simulink model "ReactionPendulum_Simulation_Model"  (R2024b)
settings: Solver=ode23  StartTime=0.0  StopTime=T_final  MaxStep=1e-2  RelTol=1e-3
values from neighbouring files (symbols this model uses):
  Control_Gain = 1.3    [PendulumControl_Mamdani_ver2.m]
  fi_pend0 = deg2rad(30)    [PendulumControl_Mamdani_ver2.m]
undefined symbols (not defined in the file or in its folder): fi_dc0, g, J_dc, J_pend, K, kr, kt, omega_dc0, omega_pend0, R_dc, U, uc_dc, uc_pend, uv_dc, uv_pend
libraries: fuzblock x1
settings Model: Creator=Student  LastModifiedBy=Paweł Wiktor
settings SolverCC: ZeroCrossAlgorithm=Adaptive  AlgebraicLoopSolver=TrustRegion
settings DataIOCC: ReturnWorkspaceOutputs=off
settings DebuggingCC: IgnoredZcDiagnostic=none  UnconnectedInputMsg=warning  UnconnectedOutputMsg=warning  UnconnectedLineMsg=warning  ArithmeticOperatorsInVariantConditions=warning
settings ModelReferenceCC: EnableRefExpFcnMdlSchedulingChecks=on
settings SFSimCC: CustomCodeUndefinedFunction=UseInterfaceOnly
settings RTWCC: GPUComputeCapability=3.5

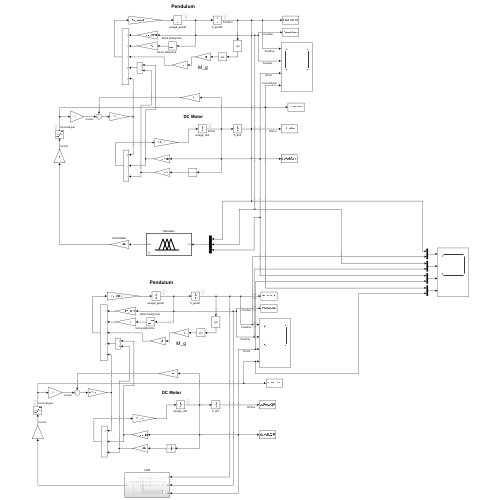
[thumbnail: Simulink's stored preview of the top-level diagram]
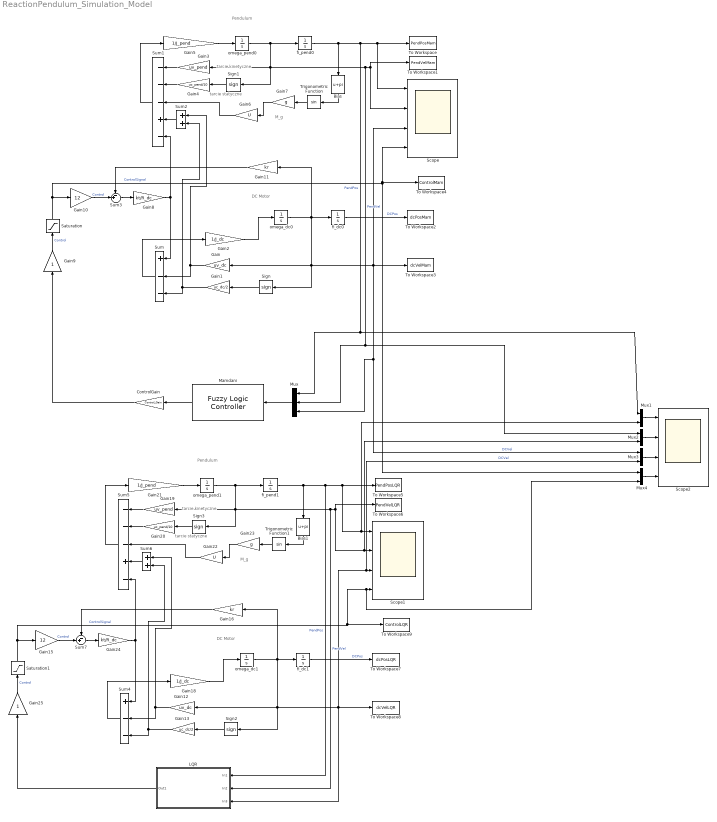
== system ReactionPendulum_Simulation_Model ==
  note: DC Motor
  note: M_g
  note: tarcie kinetyczne
  note: tarcie statyczne
  note: Pendulum
  note: DC Motor
  note: tarcie kinetyczne
  note: Pendulum
  note: tarcie statyczne
  note: M_g
  Bias : Bias  Bias=pi  SaturateOnIntegerOverflow=off
  Bias1 : Bias  Bias=pi  SaturateOnIntegerOverflow=off
  ControlGain : Gain  Gain=Control_Gain
  Gain : Gain  Gain=uv_dc
  Gain1 : Gain  Gain=uc_dc/2
  Gain10 : Gain  Gain=12
  Gain11 : Gain  Gain=kr
  Gain12 : Gain  Gain=uv_dc
  Gain13 : Gain  Gain=uc_dc/2
  Gain15 : Gain  Gain=12
  Gain16 : Gain  Gain=kr
  Gain18 : Gain  Gain=1/J_dc
  Gain19 : Gain  Gain=uv_pend
  Gain2 : Gain  Gain=1/J_dc
  Gain20 : Gain  Gain=uc_pend/10
  Gain21 : Gain  Gain=1/J_pend
  Gain22 : Gain  Gain=U
  Gain23 : Gain  Gain=g
  Gain24 : Gain  Gain=kt/R_dc
  Gain25 : Gain
  Gain3 : Gain  Gain=uv_pend
  Gain4 : Gain  Gain=uc_pend/10
  Gain5 : Gain  Gain=1/J_pend
  Gain6 : Gain  Gain=U
  Gain7 : Gain  Gain=g
  Gain8 : Gain  Gain=kt/R_dc
  Gain9 : Gain
  LQR : Subsystem
  Mamdani : fuzblock/Fuzzy Logic  Controller  FIS=fisMam_ver3  OutputSampleNumber=101  DataType=double  FuzzifiedInputs=off  RuleFiringStrengths=off  RuleOutputs=off  AggregatedOutputs=off  SimulateUsing=Interpreted execution  OutOfRangeInputValueMessage=warning  NoRuleFiredMessage=warning  EmptyOutputFuzzySetMessage=warning
  Mux : Mux  Inputs=3
  Mux{1..4} (4 alike) : Mux  Inputs=2
  Saturation : Saturate  UpperLimit=1  LowerLimit=-1
  Saturation1 : Saturate  UpperLimit=1  LowerLimit=-1
  Scope : Scope  NumInputPorts=4
  Scope1 : Scope  NumInputPorts=4
  Scope2 : Scope  NumInputPorts=4
  Sign{,1..3} (4 alike) : Signum  ZeroCross=off
  Sum : Sum  Inputs=+--
  Sum1 : Sum  Inputs=---+-
  Sum2 : Sum
  Sum3 : Sum  Inputs=-+|
  Sum4 : Sum  Inputs=+--
  Sum5 : Sum  Inputs=---+-
  Sum6 : Sum
  Sum7 : Sum  Inputs=-+|
  To Workspace : ToWorkspace  VariableName=PendPosMam  SaveFormat=Structure With Time  SampleTime=-1
  To Workspace1 : ToWorkspace  VariableName=PendVelMam  SaveFormat=Structure With Time  SampleTime=-1
  To Workspace2 : ToWorkspace  VariableName=dcPosMam  SaveFormat=Structure With Time  SampleTime=-1
  To Workspace3 : ToWorkspace  VariableName=dcVelMam  SaveFormat=Structure With Time  SampleTime=-1
  To Workspace4 : ToWorkspace  VariableName=ControlMam  SaveFormat=Structure With Time  SampleTime=-1
  To Workspace5 : ToWorkspace  VariableName=PendPosLQR  SaveFormat=Structure With Time  SampleTime=-1
  To Workspace6 : ToWorkspace  VariableName=PendVelLQR  SaveFormat=Structure With Time  SampleTime=-1
  To Workspace7 : ToWorkspace  VariableName=dcPosLQR  SaveFormat=Structure With Time  SampleTime=-1
  To Workspace8 : ToWorkspace  VariableName=dcVelLQR  SaveFormat=Structure With Time  SampleTime=-1
  To Workspace9 : ToWorkspace  VariableName=ControlLQR  SaveFormat=Structure With Time  SampleTime=-1
  Trigonometric Function : Trigonometry
  Trigonometric Function1 : Trigonometry
  fi_dc0 : Integrator  InitialCondition=fi_dc0
  fi_dc1 : Integrator  InitialCondition=fi_dc0
  fi_pend0 : Integrator  InitialCondition=fi_pend0
  fi_pend1 : Integrator  InitialCondition=fi_pend0
  omega_dc0 : Integrator  InitialCondition=omega_dc0
  omega_dc1 : Integrator  InitialCondition=omega_dc0
  omega_pend0 : Integrator  InitialCondition=omega_pend0
  omega_pend1 : Integrator  InitialCondition=omega_pend0
  wires:
  Bias/1 -> Trigonometric Function/1
  omega_pend0/1 -> Sign1/1, Mux2/1, Mux/2, To Workspace1/1, Scope/2, Gain3/1, fi_pend0/1  "PendVel"
  Gain4/1 -> Sum1/2
  Sum2/1 -> Sum1/4
  Gain11/1 -> Sum3/1
  Sum/1 -> Gain2/1
  Gain8/1 -> Sum1/5, Sum/1
  Gain3/1 -> Sum1/1
  Trigonometric Function/1 -> Gain7/1
  Sign1/1 -> Gain4/1
  Saturation/1 -> Scope/4, To Workspace4/1, Mux4/1, Gain10/1  "ControlSignal"
  Sign/1 -> Gain1/1
  Gain/1 -> Sum/2, Sum2/1
  Sum1/1 -> Gain5/1
  Gain5/1 -> omega_pend0/1
  Gain1/1 -> Sum/3, Sum2/2
  Gain10/1 -> Sum3/2  "Control"
  Gain6/1 -> Sum1/3
  Sum3/1 -> Gain8/1
  Gain2/1 -> omega_dc0/1
  Gain9/1 -> Saturation/1  "Control"
  fi_dc0/1 -> To Workspace2/1  "DCPos"
  Gain7/1 -> Gain6/1
  Mux/1 -> Mamdani/1
  ControlGain/1 -> Gain9/1
  Mamdani/1 -> ControlGain/1
  fi_pend1/1 -> LQR/1(In1), Mux1/2, Scope1/1, To Workspace5/1, Bias1/1  "PendPos"
  Sum4/1 -> Gain18/1
  Bias1/1 -> Trigonometric Function1/1
  Gain20/1 -> Sum5/2
  Gain25/1 -> Saturation1/1  "Control"
  Trigonometric Function1/1 -> Gain23/1
  Gain18/1 -> omega_dc1/1
  Gain15/1 -> Sum7/2  "Control"
  omega_pend1/1 -> Sign3/1, LQR/2(In2), To Workspace6/1, Mux2/2, Scope1/2, Gain19/1, fi_pend1/1  "PendVel"
  Sum7/1 -> Gain24/1
  Gain21/1 -> omega_pend1/1
  LQR/1(Out1) -> Gain25/1
  Saturation1/1 -> Mux4/2, Scope1/4, To Workspace9/1, Gain15/1  "ControlSignal"
  Gain16/1 -> Sum7/1
  Sum6/1 -> Sum5/4
  Gain12/1 -> Sum4/2, Sum6/1
  Sign2/1 -> Gain13/1
  Gain23/1 -> Gain22/1
  omega_dc1/1 -> Gain16/1, fi_dc1/1, Mux3/2, Scope1/3, To Workspace8/1, LQR/3(In3), Sign2/1, Gain12/1  "DCVel"
  Sum5/1 -> Gain21/1
  fi_dc1/1 -> To Workspace7/1  "DCPos"
  Gain24/1 -> Sum5/5, Sum4/1
  Gain22/1 -> Sum5/3
  Gain13/1 -> Sum4/3, Sum6/2
  Sign3/1 -> Gain20/1
  Gain19/1 -> Sum5/1
  Mux1/1 -> Scope2/1
  Mux2/1 -> Scope2/2
  Mux3/1 -> Scope2/3
  Mux4/1 -> Scope2/4
  fi_pend0/1 -> Mux1/1, Mux/1, Scope/1, To Workspace/1, Bias/1  "PendPos"
  omega_dc0/1 -> Gain11/1, fi_dc0/1, Scope/3, To Workspace3/1, Mux3/1, Mux/3, Sign/1, Gain/1  "DCVel"

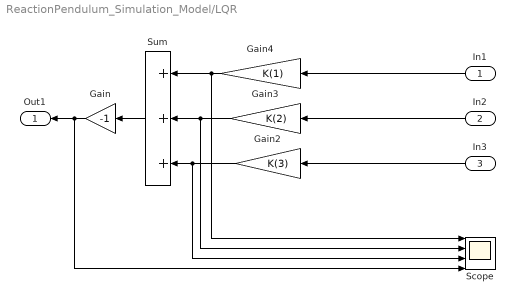
== system ReactionPendulum_Simulation_Model/LQR ==
  In1 : Inport
  In2 : Inport  Port=2
  In3 : Inport  Port=3
  Gain : Gain  Gain=-1
  Gain2 : Gain  Gain=K(3)
  Gain3 : Gain  Gain=K(2)
  Gain4 : Gain  Gain=K(1)
  Scope : Scope  NumInputPorts=4
  Sum : Sum  Inputs=+++
  Out1 : Outport  VectorParamsAs1DForOutWhenUnconnected=off
  wires:
  In1/1 -> Gain4/1
  In2/1 -> Gain3/1
  In3/1 -> Gain2/1
  Gain2/1 -> Scope/3, Sum/3
  Gain3/1 -> Scope/2, Sum/2
  Gain4/1 -> Scope/1, Sum/1
  Sum/1 -> Gain/1
  Gain/1 -> Scope/4, Out1/1
